simulink model "sim_PEG_2dim"  (R2022b)
settings: Solver=ode4  StartTime=0.0  StopTime=StopTime  FixedStep=dt  RelTol=1e-3
values from neighbouring files (symbols this model uses):
  a1_t = 0    [init_fdm.m]
  phi1_t = 0    [init_fdm.m]
  psi1 = 0    [init_fdm.m]
  psi1_t = 2*pi * (rand - 0.5)    [init_fdm.m]
  v1 = 60    [init_fdm.m]
  v1_t = 60    [init_fdm.m]
  x1 = 0    [init_fdm.m]
  x1_t = radius * cos(angle)    [init_fdm.m]
  y1 = 0    [init_fdm.m]
  y1_t = radius * sin(angle)    [init_fdm.m]
undefined symbols (not defined in the file or in its folder): DiscIntNeverNeededParam
settings Model: SimulationMode=accelerator  Creator=ykj  LastModifiedBy=ykj

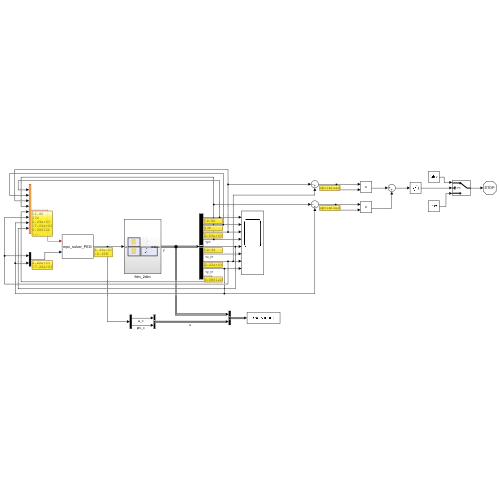
[thumbnail: Simulink's stored preview of the top-level diagram]
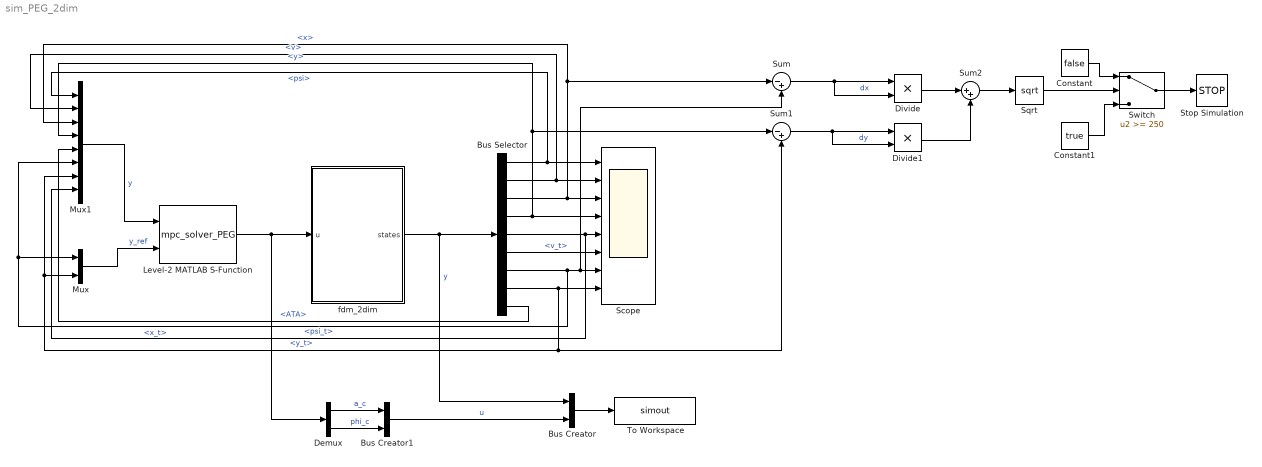
== system sim_PEG_2dim ==
  Bus Creator : BusCreator  Inputs=2
  Bus Creator1 : BusCreator  Inputs=2
  Bus Selector : BusSelector  OutputSignals=psi,v,x,y,psi_t,v_t,x_t,y_t,ATA
  Constant : Constant  Value=false  OutDataTypeStr=boolean
  Constant1 : Constant  Value=true  OutDataTypeStr=boolean
  Demux : Demux  Outputs=2
  Divide : Product  Inputs=**
  Divide1 : Product  Inputs=**
  Level-2 MATLAB S-Function : M-S-Function  FunctionName=mpc_solver_PEG
  Mux : Mux  Inputs=2
  Mux1 : Mux  Inputs=8
  Scope : Scope  NumInputPorts=8
  Sqrt : Sqrt
  Stop Simulation : Stop
  Sum : Sum  Inputs=|-+
  Sum1 : Sum  Inputs=|-+
  Sum2 : Sum  Inputs=|++
  Switch : Switch  Threshold=250  SaturateOnIntegerOverflow=off  InputSameDT=off
  To Workspace : ToWorkspace  VariableName=simout  SaveFormat=Timeseries  SampleTime=-1
  fdm_2dim : Subsystem
  wires:
  fdm_2dim/1(states) -> Bus Creator/1, Bus Selector/1  "y"
  Mux/1 -> Level-2 MATLAB S-Function/2  "y_ref"
  Bus Selector/1 -> Scope/1, Mux1/1  "<psi>"
  Bus Selector/3 -> Scope/3, Mux1/3, Sum/1  "<x>"
  Bus Selector/4 -> Scope/4, Mux1/4, Sum1/1  "<y>"
  Bus Selector/5 -> Mux1/8, Scope/5  "<psi_t>"
  Bus Selector/7 -> Mux1/6, Mux/1, Scope/7, Sum/2  "<x_t>"
  Bus Selector/8 -> Mux1/7, Mux/2, Sum1/2, Scope/8  "<y_t>"
  Level-2 MATLAB S-Function/1 -> Demux/1, fdm_2dim/1(u)
  Bus Selector/2 -> Scope/2, Mux1/2  "<v>"
  Bus Selector/6 -> Scope/6  "<v_t>"
  Mux1/1 -> Level-2 MATLAB S-Function/1  "y"
  Bus Creator/1 -> To Workspace/1
  Demux/1 -> Bus Creator1/1  "a_c"
  Demux/2 -> Bus Creator1/2  "phi_c"
  Bus Creator1/1 -> Bus Creator/2  "u"
  Bus Selector/9 -> Mux1/5  "<ATA>"
  Switch/1 -> Stop Simulation/1
  Sum/1 -> Divide/2, Divide/1  "dx"
  Sum1/1 -> Divide1/2, Divide1/1  "dy"
  Sum2/1 -> Sqrt/1
  Divide/1 -> Sum2/1
  Divide1/1 -> Sum2/2
  Sqrt/1 -> Switch/2
  Constant/1 -> Switch/1
  Constant1/1 -> Switch/3

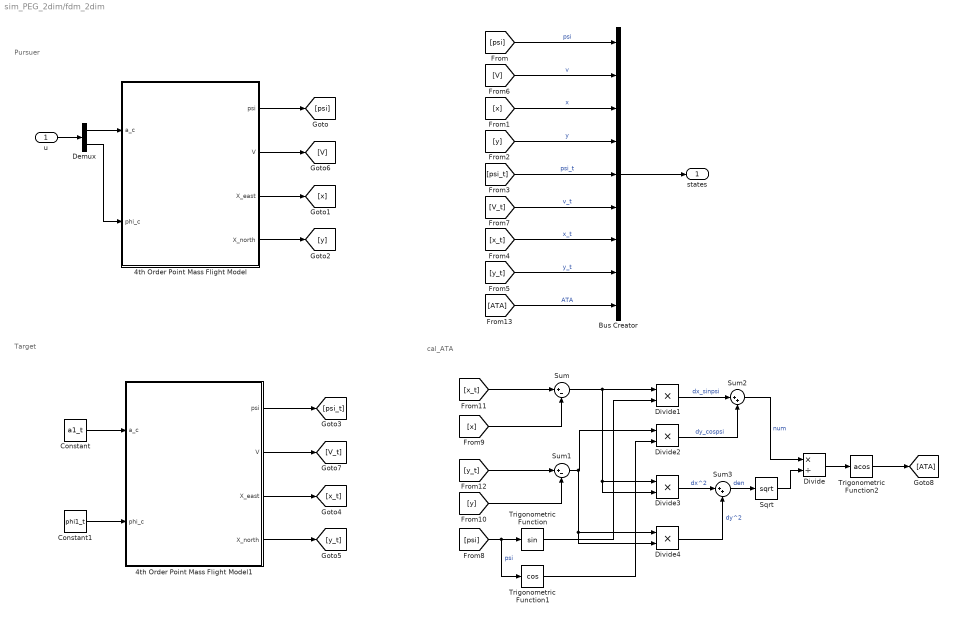
== system sim_PEG_2dim/fdm_2dim ==
  note: cal_ATA
  note: Pursuer
  note: Target
  u : Inport
  4th Order Point Mass Flight Model : Subsystem  mask{psi0=psi1, v0=v1, x0=x1, y0=y1}
      mask prompts: psi0 "Initial heading angle"; v0 "Initial airspeed"; x0 "Initial east position"; y0 "Initial north position"
      mask Display:
      | port_label('input',1,'\deltav_c(m/s^2)','texmode','on');
      | port_label('input',2,'\Phi_c(rad)','texmode','on');
      | port_label('output',1,'\Psi(rad)','texmode','on');
      | port_label('output',2,'V(m/s)','texmode','on');
      | port_label('output',3,'X_{East}(m)','texmode','on');
      | port_label('output',4,'X_{North}(m)','texmode','on');
      | text(0.5,0.5-0.08,'4th Order Point Mass','horizontalAlignment','center')
      | text(0.5,0.5+0.08,'Coordinated Flight in x-y plane','horizontalAlignment','center')
  4th Order Point Mass Flight Model1 : Subsystem  mask{psi0=psi1_t, v0=v1_t, x0=x1_t, y0=y1_t}
      mask prompts: psi0 "Initial heading angle"; v0 "Initial airspeed"; x0 "Initial east position"; y0 "Initial north position"
      mask Display:
      | port_label('input',1,'\deltav_c(m/s^2)','texmode','on');
      | port_label('input',2,'\Phi_c(rad)','texmode','on');
      | port_label('output',1,'\Psi(rad)','texmode','on');
      | port_label('output',2,'V(m/s)','texmode','on');
      | port_label('output',3,'X_{East}(m)','texmode','on');
      | port_label('output',4,'X_{North}(m)','texmode','on');
      | text(0.5,0.5-0.08,'4th Order Point Mass','horizontalAlignment','center')
      | text(0.5,0.5+0.08,'Coordinated Flight in x-y plane','horizontalAlignment','center')
  Bus Creator : BusCreator  Inputs=9
  Constant : Constant  Value=a1_t
  Constant1 : Constant  Value=phi1_t
  Demux : Demux  Outputs=2
  Divide : Product  Inputs=*/
  Divide{1..4} (4 alike) : Product  Inputs=**
  Sqrt : Sqrt
  Sum : Sum  Inputs=|+-
  Sum1 : Sum  Inputs=|+-
  Sum2 : Sum  Inputs=|++
  Sum3 : Sum  Inputs=|++
  Trigonometric Function : Trigonometry
  Trigonometric Function1 : Trigonometry  Operator=cos
  Trigonometric Function2 : Trigonometry  Operator=acos
  states : Outport
  wires:
  Constant/1 -> 4th Order Point Mass Flight Model1/1(a_c)
  Constant1/1 -> 4th Order Point Mass Flight Model1/2(phi_c)
  4th Order Point Mass Flight Model/3(X_east) -> [x]
  4th Order Point Mass Flight Model/1(psi) -> [psi]
  4th Order Point Mass Flight Model/4(X_north) -> [y]
  4th Order Point Mass Flight Model1/3(X_east) -> [x_t]
  4th Order Point Mass Flight Model1/1(psi) -> [psi_t]
  4th Order Point Mass Flight Model1/4(X_north) -> [y_t]
  Bus Creator/1 -> states/1
  [psi] -> Bus Creator/1  "psi"
  u/1 -> Demux/1
  Demux/1 -> 4th Order Point Mass Flight Model/1(a_c)
  Demux/2 -> 4th Order Point Mass Flight Model/2(phi_c)
  4th Order Point Mass Flight Model/2(V) -> [V]
  4th Order Point Mass Flight Model1/2(V) -> [V_t]
  [V] -> Bus Creator/2  "v"
  [x] -> Bus Creator/3  "x"
  [y] -> Bus Creator/4  "y"
  [psi_t] -> Bus Creator/5  "psi_t"
  [V_t] -> Bus Creator/6  "v_t"
  [x_t] -> Bus Creator/7  "x_t"
  [y_t] -> Bus Creator/8  "y_t"
  [x] -> Sum/2
  [x_t] -> Sum/1
  [y_t] -> Sum1/1
  [y] -> Sum1/2
  Sum/1 -> Divide3/2, Divide3/1, Divide1/1
  [ATA] -> Bus Creator/9  "ATA"
  Divide/1 -> Trigonometric Function2/1
  Sum1/1 -> Divide4/1, Divide4/2, Divide2/1
  [psi] -> Trigonometric Function1/1, Trigonometric Function/1  "psi"
  Trigonometric Function1/1 -> Divide2/2
  Trigonometric Function/1 -> Divide1/2
  Trigonometric Function2/1 -> [ATA]
  Divide1/1 -> Sum2/1  "dx_sinpsi"
  Divide2/1 -> Sum2/2  "dy_cospsi"
  Sum2/1 -> Divide/1  "num"
  Divide3/1 -> Sum3/1  "dx^2"
  Sum3/1 -> Sqrt/1  "den"
  Divide4/1 -> Sum3/2  "dy^2"
  Sqrt/1 -> Divide/2

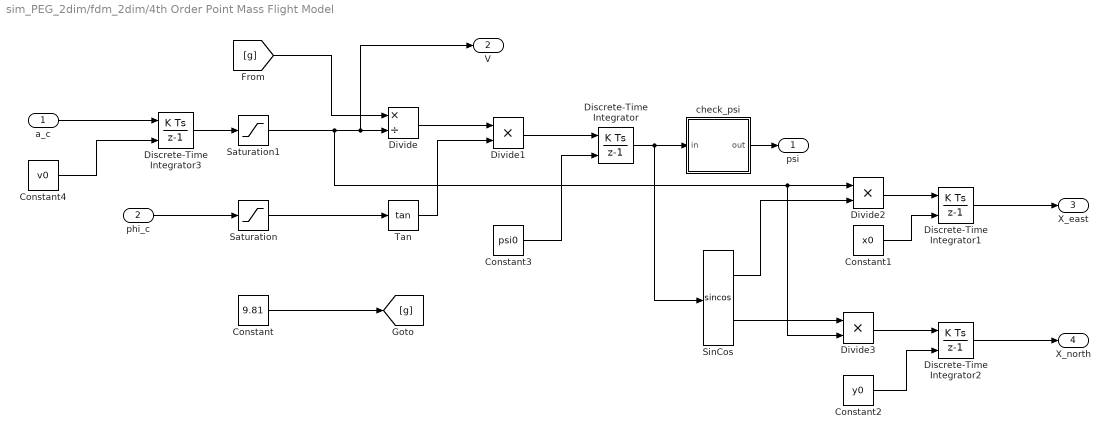
== system sim_PEG_2dim/fdm_2dim/4th Order Point Mass Flight Model ==
  a_c : Inport
  phi_c : Inport  Port=2
  Constant : Constant  Value=9.81
  Constant1 : Constant  Value=x0
  Constant2 : Constant  Value=y0
  Constant3 : Constant  Value=psi0
  Constant4 : Constant  Value=v0
  Discrete-Time Integrator : DiscreteIntegrator  InitialConditionSource=external  InitialCondition=psi0  SampleTime=-1  ICPrevOutput=DiscIntNeverNeededParam  ICPrevScaledInput=DiscIntNeverNeededParam
  Discrete-Time Integrator1 : DiscreteIntegrator  InitialConditionSource=external  InitialCondition=x0  SampleTime=-1  ICPrevOutput=DiscIntNeverNeededParam  ICPrevScaledInput=DiscIntNeverNeededParam
  Discrete-Time Integrator2 : DiscreteIntegrator  InitialConditionSource=external  InitialCondition=y0  SampleTime=-1  ICPrevOutput=DiscIntNeverNeededParam  ICPrevScaledInput=DiscIntNeverNeededParam
  Discrete-Time Integrator3 : DiscreteIntegrator  InitialConditionSource=external  InitialCondition=v0  SampleTime=-1  ICPrevOutput=DiscIntNeverNeededParam  ICPrevScaledInput=DiscIntNeverNeededParam
  Divide : Product  Inputs=*/
  Divide1 : Product  Inputs=**
  Divide2 : Product  Inputs=**
  Divide3 : Product  Inputs=**
  Saturation : Saturate  UpperLimit=30/57.3  LowerLimit=-30/57.3
  Saturation1 : Saturate  UpperLimit=130  LowerLimit=60
  SinCos : Trigonometry  Operator=sincos
  Tan : Trigonometry  Operator=tan
  check_psi : Stateflow chart  TreatAsAtomicUnit=on
  psi : Outport
  V : Outport  Port=2
  X_east : Outport  Port=3
  X_north : Outport  Port=4
  wires:
  phi_c/1 -> Saturation/1
  a_c/1 -> Discrete-Time Integrator3/1
  Constant/1 -> [g]
  Saturation1/1 -> V/1, Divide/2, Divide2/1, Divide3/2
  [g] -> Divide/1
  Divide/1 -> Divide1/1
  Saturation/1 -> Tan/1
  Tan/1 -> Divide1/2
  Divide1/1 -> Discrete-Time Integrator/1
  Discrete-Time Integrator/1 -> check_psi/1(in), SinCos/1
  SinCos/2 -> Divide3/1
  Divide3/1 -> Discrete-Time Integrator2/1
  Discrete-Time Integrator1/1 -> X_east/1
  Discrete-Time Integrator2/1 -> X_north/1
  Divide2/1 -> Discrete-Time Integrator1/1
  SinCos/1 -> Divide2/2
  Constant1/1 -> Discrete-Time Integrator1/2
  Constant2/1 -> Discrete-Time Integrator2/2
  Constant3/1 -> Discrete-Time Integrator/2
  Discrete-Time Integrator3/1 -> Saturation1/1
  Constant4/1 -> Discrete-Time Integrator3/2
  check_psi/1(out) -> psi/1

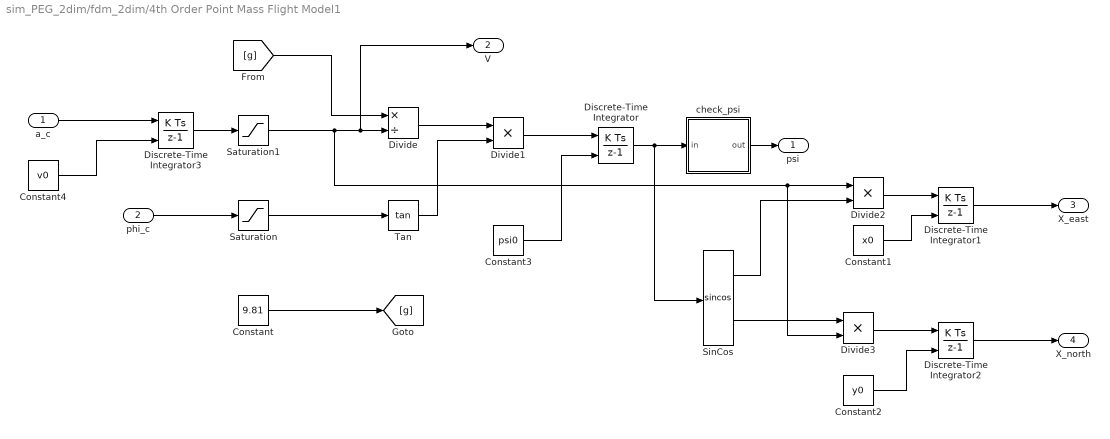
== system sim_PEG_2dim/fdm_2dim/4th Order Point Mass Flight Model1 ==
  a_c : Inport
  phi_c : Inport  Port=2
  Constant : Constant  Value=9.81
  Constant1 : Constant  Value=x0
  Constant2 : Constant  Value=y0
  Constant3 : Constant  Value=psi0
  Constant4 : Constant  Value=v0
  Discrete-Time Integrator : DiscreteIntegrator  InitialConditionSource=external  InitialCondition=psi0  SampleTime=-1  ICPrevOutput=DiscIntNeverNeededParam  ICPrevScaledInput=DiscIntNeverNeededParam
  Discrete-Time Integrator1 : DiscreteIntegrator  InitialConditionSource=external  InitialCondition=x0  SampleTime=-1  ICPrevOutput=DiscIntNeverNeededParam  ICPrevScaledInput=DiscIntNeverNeededParam
  Discrete-Time Integrator2 : DiscreteIntegrator  InitialConditionSource=external  InitialCondition=y0  SampleTime=-1  ICPrevOutput=DiscIntNeverNeededParam  ICPrevScaledInput=DiscIntNeverNeededParam
  Discrete-Time Integrator3 : DiscreteIntegrator  InitialConditionSource=external  InitialCondition=v0  SampleTime=-1  ICPrevOutput=DiscIntNeverNeededParam  ICPrevScaledInput=DiscIntNeverNeededParam
  Divide : Product  Inputs=*/
  Divide1 : Product  Inputs=**
  Divide2 : Product  Inputs=**
  Divide3 : Product  Inputs=**
  Saturation : Saturate  UpperLimit=30/57.3  LowerLimit=-30/57.3
  Saturation1 : Saturate  UpperLimit=130  LowerLimit=60
  SinCos : Trigonometry  Operator=sincos
  Tan : Trigonometry  Operator=tan
  check_psi : Stateflow chart  TreatAsAtomicUnit=on
  psi : Outport
  V : Outport  Port=2
  X_east : Outport  Port=3
  X_north : Outport  Port=4
  wires:
  phi_c/1 -> Saturation/1
  a_c/1 -> Discrete-Time Integrator3/1
  Constant/1 -> [g]
  Saturation1/1 -> V/1, Divide/2, Divide2/1, Divide3/2
  [g] -> Divide/1
  Divide/1 -> Divide1/1
  Saturation/1 -> Tan/1
  Tan/1 -> Divide1/2
  Divide1/1 -> Discrete-Time Integrator/1
  Discrete-Time Integrator/1 -> check_psi/1(in), SinCos/1
  SinCos/2 -> Divide3/1
  Divide3/1 -> Discrete-Time Integrator2/1
  Discrete-Time Integrator1/1 -> X_east/1
  Discrete-Time Integrator2/1 -> X_north/1
  Divide2/1 -> Discrete-Time Integrator1/1
  SinCos/1 -> Divide2/2
  Constant1/1 -> Discrete-Time Integrator1/2
  Constant2/1 -> Discrete-Time Integrator2/2
  Constant3/1 -> Discrete-Time Integrator/2
  Discrete-Time Integrator3/1 -> Saturation1/1
  Constant4/1 -> Discrete-Time Integrator3/2
  check_psi/1(out) -> psi/1

== stateflow chart sim_PEG_2dim/fdm_2dim/4th Order Point Mass Flight Model1/check_psi ==
  (default) -> (junction 1)
  (junction 1) -> (junction 3) [order 1] : [in < -pi]
  (junction 1) -> (junction 7) [order 2]
  (junction 3) -> (junction 5) : {out = in + 2*pi;}
  (junction 7) -> (junction 9) [order 1] : [in > pi]
  (junction 7) -> (junction 14) [order 2] : {out=in;}
  (junction 9) -> (junction 11) : {out = in-2*pi;}
  (junction 11) -> (junction 14)
  (junction 5) -> (junction 11)
  (junction 14) -> (junction 17)
  data: out output; in input

== stateflow chart sim_PEG_2dim/fdm_2dim/4th Order Point Mass Flight Model/check_psi ==
  (default) -> (junction 1)
  (junction 1) -> (junction 3) [order 1] : [in < -pi]
  (junction 1) -> (junction 7) [order 2]
  (junction 3) -> (junction 5) : {out = in + 2*pi;}
  (junction 7) -> (junction 9) [order 1] : [in > pi]
  (junction 7) -> (junction 14) [order 2] : {out=in;}
  (junction 9) -> (junction 11) : {out = in-2*pi;}
  (junction 11) -> (junction 14)
  (junction 5) -> (junction 11)
  (junction 14) -> (junction 17)
  data: out output; in input
